simulink model "sampleModel1697"  (R2023a)
settings: Solver=VariableStepAuto  StartTime=0.0  StopTime=10.0  RelTol=1e-3
libraries: hdlsllib x6
settings Model: Creator=user1  LastModifiedBy=user1

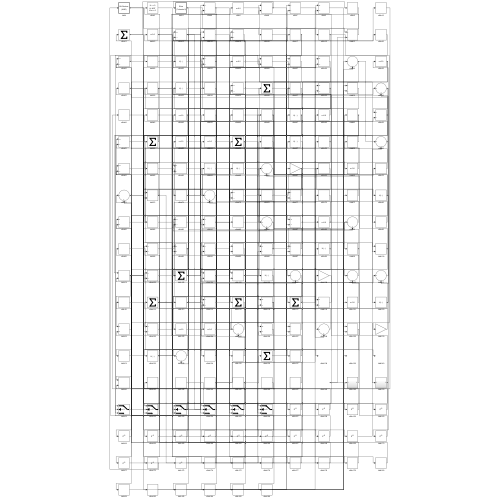
[thumbnail: Simulink's stored preview of the top-level diagram]
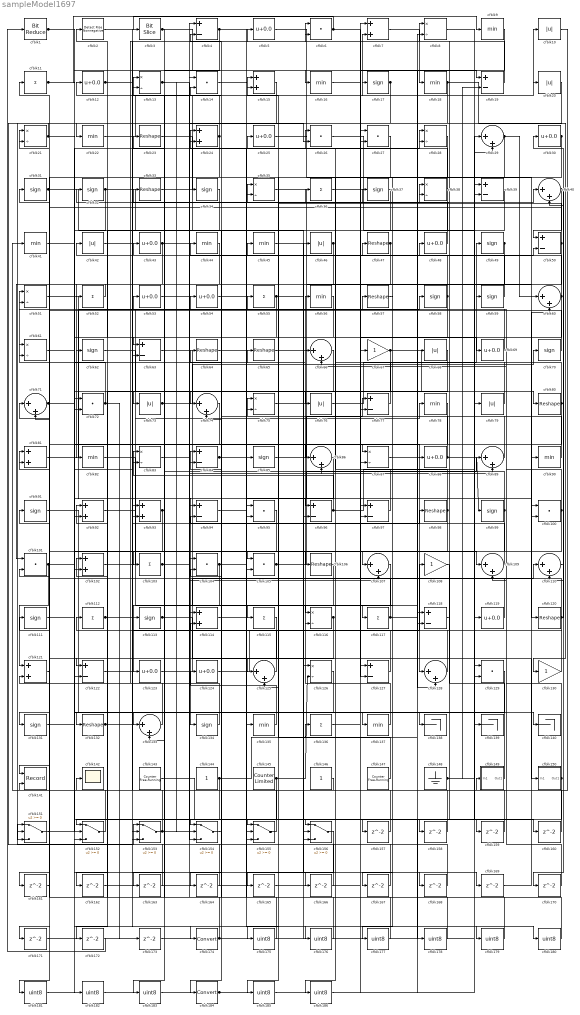
== system sampleModel1697 ==
  cfblk1 : hdlsllib/Logic and Bit Operations/Bit Reduce  mode=AND
  cfblk{10,20,42,46,68,73,76,79} (8 alike) : Abs  SaturateOnIntegerOverflow=off
  cfblk{6,14,26..27,72,95,100..101,104..105,129} (11 alike) : DotProduct  OutDataTypeStr=Inherit: Inherit via internal rule
  cfblk{7,15,24,81,92..93,102,114,121} (9 alike) : Sum
  cfblk{11,36,52,55,103,112,115,117,136} (9 alike) : Sum  Inputs=+
  cfblk{23,33,47,57,64..65,80,98,106,120,132} (11 alike) : Reshape
  cfblk{29,40,60,66,71,74,86,89,107,109..110,125,128,133} (14 alike) : Sum  Inputs=|++
  cfblk108 : Gain
  cfblk{17,31..32,34,37,49,58..59,62,70,85,91,99,111,113,131,134} (17 alike) : Signum
  cfblk{8,13,21,28,35,38,51,61,75,83,87,116,126} (13 alike) : Product  Inputs=*/  RndMeth=Zero  SaturateOnIntegerOverflow=on
  cfblk{4,19,39,50,63,77,84,94,96..97,118,122,127} (13 alike) : Sum  Inputs=+-
  cfblk{5,12,25,30,43,48,53..54,69,88,119,123..124} (13 alike) : Bias  Bias=0.0  SaturateOnIntegerOverflow=off
  cfblk130 : Gain
  cfblk{9,16,18,22,41,44..45,56,78,82,90,135,137} (13 alike) : MinMax
  cfblk138 : Terminator
  cfblk139 : Terminator
  cfblk140 : Terminator
  cfblk141 : Record  FileSettingsInternal="{\"entries\":[{\"content\":{\"excelSettings\":{\"content\":{},\"type\":\"Streamout.ExcelSettings\"}},\"type\":\"Streamout.FileSettingStorage\",\"uuid\":\"\"}],\"packageUris\":[\"http:\\/\\/schema.mathworks.com\\/mf0\\/streamout_blocks\\/R2020a\"],\"version\":\"1.0\"}"  Layout=[1 1]  SignalsInternal="{\"entries\":[{\"content\":{\"signals\":[{\"content\":{\"blockPath\":[],\"dimensions\":[1],\"domain\":\"\",\"lineColor\":\"#a2142f\",\"plots\":[1],\"port\":1,\"signalID\":3036,\"signalName\":\"XY Graph:1\"},\"type\":\"RecordBlkView.Signal\",\"uuid\":\"\"},{\"content\":{\"blockPath\":[],\"dimensions\":[1],\"domain\":\"\",\"lineColor\":\"#139fff\",\"plots\":[1],\"port\":2,\"signalID\":3039,\"signalName\":\"XY Graph:2\"},\"type\":\"RecordBlkView.Signal\",\"uuid\":\"\"}]},\"type\":\"RecordBlkView.InputSignals\",\"uuid\":\"\"}],\"packageUris\":[\"http:\\/\\/schema.mathworks.com\\/mf0\\/streamout_blocks\\/R2020a\"],\"version\":\"1.0\"}"  VisualizationBindings="{\"xyplotplugin\":{\"info\":[{\"series\":[{\"bindingParametersList\":[{\"parameter\":\"X-Axis\",\"signalID\":3036,\"signalName\":\"XY Graph:1\"},{\"parameter\":\"Y-Axis\",\"signalID\":3039,\"signalName\":\"XY Graph:2\"}],\"seriesID\":38226}],\"subplotID\":1}]}}"  CompatibilityTag=XY  st=-1
  cfblk142 : Scope
  cfblk143 : hdlsllib/Sources/Counter Free-Running  NumBits=16  tsamp=-1
  cfblk144 : Constant  SampleTime=-1
  cfblk145 : hdlsllib/Sources/Counter Limited  uplimit=7  tsamp=-1
  cfblk146 : Constant  SampleTime=-1
  cfblk147 : hdlsllib/Sources/Counter Free-Running  NumBits=16  tsamp=-1
  cfblk148 : Ground
  cfblk149 : Subsystem
      settings: LibrarySourceBlock=|
      | hdlsllib/Ports &
      | Subsystems/Subsystem
  cfblk150 : Subsystem
      settings: LibrarySourceBlock=|
      | hdlsllib/Ports &
      | Subsystems/Subsystem
  cfblk{151..156} (6 alike) : Switch  SaturateOnIntegerOverflow=off  InputSameDT=off
  cfblk{157..173} (17 alike) : Delay  SampleTime=1
  cfblk174 : DataTypeConversion  SaturateOnIntegerOverflow=off  RndMeth=Floor
  cfblk{175..183,185..186} (11 alike) : DataTypeConversion  OutDataTypeStr=uint8  SaturateOnIntegerOverflow=off  RndMeth=Floor
  cfblk184 : DataTypeConversion  SaturateOnIntegerOverflow=off  RndMeth=Floor
  cfblk2 : hdlsllib/Logic and Bit Operations/Detect Rise Nonnegative  vinit=0  OutDataTypeStr=boolean
  cfblk3 : hdlsllib/Logic and Bit Operations/Bit Slice  lidx=7  ridx=0
  cfblk67 : Gain
  wires:
  cfblk35/1 -> cfblk87/1
  cfblk104/1 -> cfblk123/1, cfblk28/1
  cfblk101/1 -> cfblk121/1, cfblk105/1, cfblk28/2, cfblk83/1
  cfblk58/1 -> cfblk25/1, cfblk105/2
  cfblk39/1 -> cfblk184/1
  cfblk29/1 -> cfblk60/1, cfblk117/1
  cfblk19/1 -> cfblk6/1
  cfblk72/1 -> cfblk51/1, cfblk173/1
  cfblk7/1 -> cfblk18/1
  cfblk98/1 -> cfblk75/1, cfblk177/1
  cfblk117/1 -> cfblk43/1, cfblk40/1
  cfblk110/1 -> cfblk30/1
  cfblk133/1 -> cfblk5/1
  cfblk30/1 -> cfblk107/1, cfblk76/1
  cfblk91/1 -> cfblk140/1
  cfblk92/1 -> cfblk57/1
  cfblk149/1(Out1) -> cfblk36/1
  cfblk81/1 -> cfblk58/1
  cfblk95/1 -> cfblk131/1
  cfblk63/1 -> cfblk115/1
  cfblk136/1 -> cfblk67/1
  cfblk59/1 -> cfblk47/1
  cfblk74/1 -> cfblk141/1
  cfblk80/1 -> cfblk44/1, cfblk53/1, cfblk170/1, cfblk171/1
  cfblk89/1 -> cfblk48/1
  cfblk137/1 -> cfblk56/1
  cfblk52/1 -> cfblk101/1
  cfblk23/1 -> cfblk126/1
  cfblk99/1 -> cfblk13/1, cfblk153/2
  cfblk123/1 -> cfblk110/1
  cfblk2/1 -> cfblk174/1
  cfblk147/1 -> cfblk55/1
  cfblk73/1 -> cfblk70/1, cfblk45/1
  cfblk67/1 -> cfblk122/1, cfblk100/1, cfblk156/1
  cfblk40/1 -> cfblk50/1, cfblk110/2
  cfblk46/1 -> cfblk133/1, cfblk125/2
  cfblk119/1 -> cfblk35/1
  cfblk86/1 -> cfblk134/1
  cfblk34/1 -> cfblk113/1
  cfblk145/1 -> cfblk126/2, cfblk155/3
  cfblk135/1 -> cfblk124/1
  cfblk69/1 -> cfblk21/1
  cfblk120/1 -> cfblk31/1, cfblk40/2, cfblk114/2
  cfblk87/1 -> cfblk128/1
  cfblk9/1 -> cfblk87/2
  cfblk51/1 -> cfblk94/1
  cfblk76/1 -> cfblk49/1
  cfblk116/1 -> cfblk125/1, cfblk161/1
  cfblk146/1 -> cfblk41/1
  cfblk100/1 -> cfblk66/2, cfblk163/1
  cfblk78/1 -> cfblk104/1
  cfblk18/1 -> cfblk130/1, cfblk151/2
  cfblk93/1 -> cfblk152/1, cfblk33/1
  cfblk49/1 -> cfblk82/1, cfblk154/3
  cfblk82/1 -> cfblk135/1
  cfblk88/1 -> cfblk99/1, cfblk12/1
  cfblk144/1 -> cfblk136/1, cfblk24/1, cfblk153/3, cfblk8/2
  cfblk11/1 -> cfblk9/1, cfblk137/1
  cfblk5/1 -> cfblk127/1
  cfblk129/1 -> cfblk132/1
  cfblk151/1 -> cfblk65/1
  cfblk113/1 -> cfblk150/1(In1), cfblk66/1
  cfblk152/1 -> cfblk141/2
  cfblk85/1 -> cfblk77/1
  cfblk4/1 -> cfblk63/1, cfblk100/2
  cfblk112/1 -> cfblk138/1, cfblk116/2, cfblk156/2
  cfblk56/1 -> cfblk155/1
  cfblk105/1 -> cfblk89/1, cfblk168/1
  cfblk124/1 -> cfblk108/1
  cfblk64/1 -> cfblk96/1
  cfblk22/1 -> cfblk10/1
  cfblk90/1 -> cfblk35/2
  cfblk75/1 -> cfblk127/2
  cfblk150/1(Out1) -> cfblk59/1, cfblk172/1
  cfblk36/1 -> cfblk128/2
  cfblk33/1 -> cfblk7/2
  cfblk153/1 -> cfblk142/1, cfblk81/1, cfblk107/2, cfblk50/2
  cfblk55/1 -> cfblk114/1, cfblk88/1
  cfblk102/1 -> cfblk78/1
  cfblk96/1 -> cfblk29/1, cfblk83/2
  cfblk43/1 -> cfblk34/1, cfblk151/3
  cfblk77/1 -> cfblk42/1
  cfblk62/1 -> cfblk80/1
  cfblk106/1 -> cfblk154/1
  cfblk109/1 -> cfblk64/1
  cfblk12/1 -> cfblk75/2, cfblk180/1
  cfblk148/1 -> cfblk119/1, cfblk19/2
  cfblk114/1 -> cfblk26/1
  cfblk127/1 -> cfblk15/1
  cfblk26/1 -> cfblk129/1
  cfblk53/1 -> cfblk4/1
  cfblk128/1 -> cfblk92/1
  cfblk155/1 -> cfblk61/1
  cfblk17/1 -> cfblk77/2, cfblk122/2
  cfblk134/1 -> cfblk61/2
  cfblk118/1 -> cfblk8/1
  cfblk50/1 -> cfblk15/2, cfblk92/2, cfblk11/1, cfblk186/1
  cfblk13/1 -> cfblk133/2, cfblk19/1, cfblk26/2, cfblk154/2
  cfblk24/1 -> cfblk13/2, cfblk183/1
  cfblk65/1 -> cfblk129/2
  cfblk3/1 -> cfblk118/1, cfblk103/1
  cfblk130/1 -> cfblk102/1
  cfblk79/1 -> cfblk54/1
  cfblk47/1 -> cfblk102/2, cfblk62/1
  cfblk48/1 -> cfblk37/1
  cfblk154/1 -> cfblk84/1
  cfblk125/1 -> cfblk4/2
  cfblk16/1 -> cfblk97/1
  cfblk32/1 -> cfblk72/2, cfblk86/2, cfblk38/2
  cfblk103/1 -> cfblk89/2, cfblk17/1
  cfblk38/1 -> cfblk52/1, cfblk74/2, cfblk24/2
  cfblk1/1 -> cfblk16/1, cfblk156/3
  cfblk15/1 -> cfblk84/2
  cfblk132/1 -> cfblk98/1, cfblk6/2
  cfblk31/1 -> cfblk85/1, cfblk169/1
  cfblk21/1 -> cfblk153/1, cfblk86/1
  cfblk41/1 -> cfblk74/1
  cfblk54/1 -> cfblk116/1
  cfblk25/1 -> cfblk90/1
  cfblk68/1 -> cfblk95/2
  cfblk84/1 -> cfblk118/2, cfblk159/1
  cfblk70/1 -> cfblk21/2
  cfblk97/1 -> cfblk32/1
  cfblk6/1 -> cfblk3/1, cfblk69/1
  cfblk121/1 -> cfblk71/1
  cfblk10/1 -> cfblk149/1(In1)
  cfblk45/1 -> cfblk120/1
  cfblk44/1 -> cfblk63/2
  cfblk94/1 -> cfblk109/1
  cfblk122/1 -> cfblk20/1
  cfblk83/1 -> cfblk106/1
  cfblk126/1 -> cfblk152/2
  cfblk107/1 -> cfblk155/2
  cfblk20/1 -> cfblk22/1
  cfblk71/1 -> cfblk93/2, cfblk73/1
  cfblk60/1 -> cfblk152/3, cfblk38/1
  cfblk61/1 -> cfblk157/1
  cfblk157/1 -> cfblk94/2
  cfblk108/1 -> cfblk158/1
  cfblk158/1 -> cfblk104/2
  cfblk159/1 -> cfblk93/1
  cfblk8/1 -> cfblk160/1
  cfblk160/1 -> cfblk72/1
  cfblk161/1 -> cfblk101/2
  cfblk115/1 -> cfblk162/1
  cfblk162/1 -> cfblk7/1
  cfblk163/1 -> cfblk51/2
  cfblk66/1 -> cfblk164/1
  cfblk164/1 -> cfblk121/2
  cfblk156/1 -> cfblk165/1
  cfblk165/1 -> cfblk96/2
  cfblk42/1 -> cfblk166/1
  cfblk166/1 -> cfblk71/2
  cfblk57/1 -> cfblk167/1
  cfblk167/1 -> cfblk151/1
  cfblk168/1 -> cfblk81/2
  cfblk169/1 -> cfblk60/2
  cfblk170/1 -> cfblk109/2
  cfblk171/1 -> cfblk29/2
  cfblk172/1 -> cfblk1/1
  cfblk173/1 -> cfblk97/2
  cfblk174/1 -> cfblk46/1, cfblk23/1, cfblk112/1
  cfblk28/1 -> cfblk175/1
  cfblk175/1 -> cfblk2/1
  cfblk14/1 -> cfblk176/1
  cfblk176/1 -> cfblk91/1
  cfblk177/1 -> cfblk14/1
  cfblk143/1 -> cfblk178/1
  cfblk178/1 -> cfblk14/2
  cfblk111/1 -> cfblk179/1
  cfblk179/1 -> cfblk95/1
  cfblk180/1 -> cfblk111/1
  cfblk27/1 -> cfblk181/1
  cfblk181/1 -> cfblk139/1
  cfblk131/1 -> cfblk182/1
  cfblk182/1 -> cfblk27/1
  cfblk183/1 -> cfblk27/2
  cfblk184/1 -> cfblk68/1, cfblk79/1
  cfblk37/1 -> cfblk185/1
  cfblk185/1 -> cfblk39/1
  cfblk186/1 -> cfblk39/2

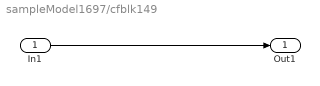
== system sampleModel1697/cfblk149 ==
  In1 : Inport
  Out1 : Outport
  wires:
  In1/1 -> Out1/1

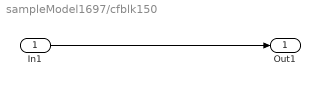
== system sampleModel1697/cfblk150 ==
  In1 : Inport
  Out1 : Outport
  wires:
  In1/1 -> Out1/1
